simulink model "state_MCP_ER0"  (R2019b)
settings: Solver=FixedStepAuto  StartTime=0.0  StopTime=100  RelTol=1e-3
InitFcn:
  | rpm=[900 1000 1100 1200 1300 1400 1500 1600 1700 1800 1900];
settings Model: Creator=victo  LastModifiedBy=victo
settings DataIOCC: SaveOutput=off  SaveTime=off

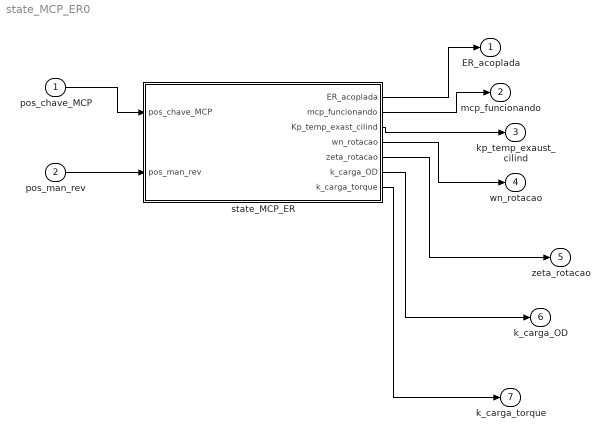
== system state_MCP_ER0 ==
  pos_chave_MCP : Inport  OutDataTypeStr=double  PortDimensions=1
  pos_man_rev : Inport  Port=2  OutDataTypeStr=double  PortDimensions=1
  state_MCP_ER : Stateflow chart  TreatAsAtomicUnit=on
  ER_acoplada : Outport  OutDataTypeStr=double  PortDimensions=1  SampleTime=[0,1]
  mcp_funcionando : Outport  Port=2  OutDataTypeStr=double  PortDimensions=1  SampleTime=[0,1]
  kp_temp_exaust_cilind : Outport  Port=3  OutDataTypeStr=double  PortDimensions=1  SampleTime=[0,1]
  wn_rotacao : Outport  Port=4  OutDataTypeStr=double  PortDimensions=1  SampleTime=[0,1]
  zeta_rotacao : Outport  Port=5  OutDataTypeStr=double  PortDimensions=1  SampleTime=[0,1]
  k_carga_OD : Outport  Port=6  OutDataTypeStr=double  PortDimensions=1  SampleTime=[0,1]
  k_carga_torque : Outport  Port=7  OutDataTypeStr=double  PortDimensions=1  SampleTime=[0,1]
  wires:
  pos_chave_MCP/1 -> state_MCP_ER/1(pos_chave_MCP)
  pos_man_rev/1 -> state_MCP_ER/2(pos_man_rev)
  state_MCP_ER/1(ER_acoplada) -> ER_acoplada/1
  state_MCP_ER/2(mcp_funcionando) -> mcp_funcionando/1
  state_MCP_ER/3(Kp_temp_exast_cilind) -> kp_temp_exaust_cilind/1
  state_MCP_ER/4(wn_rotacao) -> wn_rotacao/1
  state_MCP_ER/5(zeta_rotacao) -> zeta_rotacao/1
  state_MCP_ER/6(k_carga_OD) -> k_carga_OD/1
  state_MCP_ER/7(k_carga_torque) -> k_carga_torque/1

== stateflow chart state_MCP_ER0/state_MCP_ER ==
  state STATUS_MCP [parallel]
    settings: executionOrder=1
    state START
      entry: mcp_funcionando=1;
    state ON
      entry: mcp_funcionando=0;
    state GLOW
      entry: mcp_funcionando=0
    state OFF
      entry: mcp_funcionando=0
    (default) -> OFF
    OFF -> GLOW [order 1] : [pos_chave_MCP==-1]
    ON -> START [order 2] : [pos_chave_MCP==2]
    OFF -> ON [order 2] : [pos_chave_MCP==1]
    GLOW -> OFF : [pos_chave_MCP==0]
    START -> ON : [pos_chave_MCP==1]
    ON -> OFF [order 1] : [pos_chave_MCP==0]
  state STATUS_ER [parallel]
    settings: executionOrder=2
    state NEUTRO
      entry: Kp_temp_exast_cilind=10/1300;
      ER_acoplada=0;
      wn_rotacao=1.2;
      zeta_rotacao=0.7;
      k_carga_OD=1;
      k_carga_torque=0.67;
    state DIRETO
      entry: Kp_temp_exast_cilind=69.8/200;
      wn_rotacao=1.2;
      zeta_rotacao=0.9;
      ER_acoplada=1;
      k_carga_OD=1.2;
      k_carga_torque=1;
    state REVERSORA
      entry: Kp_temp_exast_cilind=69.8/200;
      ER_acoplada=1;
      wn_rotacao=0.5;
      zeta_rotacao=0.9;
      k_carga_OD=1.2;
      k_carga_torque=1;
    NEUTRO -> DIRETO [order 1] : [pos_man_rev==1]
    (default) -> NEUTRO
    DIRETO -> NEUTRO : [pos_man_rev==0]
    NEUTRO -> REVERSORA [order 2] : [pos_man_rev==-1]
    REVERSORA -> NEUTRO : [pos_man_rev==0]
  data: pos_chave_MCP input; pos_man_rev input; ER_acoplada output; mcp_funcionando output; Kp_temp_exast_cilind output double; wn_rotacao output; zeta_rotacao output; k_carga_OD output; k_carga_torque output
